simulink model "sliding_car"  (R2017a)
settings: Solver=VariableStepAuto  StartTime=0.0  StopTime=tf  RelTol=1e-3
values from neighbouring files (symbols this model uses):
  R = sys.descrip.syms(end-4)    [load_consts.m]
  sys = kinematic_model(sys)    [load_kin.m]
undefined symbols (not defined in the file or in its folder): a, Cp_1, Cp_2, Fz_1, Fz_2, g, Ic_33, Ii_11, Ii_21, Ii_22, Ii_31, Ii_32, Ii_33, Il_11, Il_21, Il_22, Il_31, Il_32, Il_33, Io_11, Io_21, Io_22, Io_31, Io_32, Io_33, Ir_11, Ir_21, Ir_22, Ir_31, Ir_32, Ir_33, L, Lc, mc, mi, ml, mo, mr, mu_1, mu_2, w, x0
(part 3 of 5)

== matlab function sliding_car/Vehicle/Steering automobile model/Auxiliary matrices/dA_1delta ==
  data: x input; kappa_1 input; kappa_2 input; alpha_1 input; alpha_2 input; w parameter; L parameter; R parameter; dA_1delta output
function dA_1delta = dConstraintMatrix(x, kappa_1, kappa_2, alpha_1, alpha_2, w, L, R)
%DCONSTRAINTMATRIX
%    A_1DELTA = DCONSTRAINTMATRIX(L,R,ALPHA_1,ALPHA_2,DELTA_I,DELTA_O,KAPPA_1,KAPPA_2,THETA,W)

%    This function was generated by the Symbolic Math Toolbox version 7.2.
%    16-Oct-2020 14:33:54
    
    x_pos =  x(1);
    y_pos =  x(2);
    theta =  x(3);

    delta_i = x(4);
    delta_o = x(5);

    phi_i = x(6);
    phi_l = x(7);
    phi_o = x(8);
    phi_r = x(9);

    t2 = tan(delta_i);
    t3 = 1.0./L;
    t4 = t2.*w;
    t5 = L+t4;
    t6 = 1.0./t5;
    t7 = t2.*t6;
    t8 = tan(t7);
    t9 = delta_i+theta;
    t10 = cos(t9);
    t11 = sin(t9);
    t12 = tan(alpha_1);
    t13 = cos(delta_i);
    t14 = sin(delta_i);
    t15 = t14.*w.*(1.0./2.0);
    t16 = kappa_1.*t10.*t12;
    t17 = kappa_1.*t11.*t12;
    t18 = kappa_1.*t12.*(t15-L.*t13);
    t19 = L.*t8;
    t20 = atan(t19);
    t21 = t20+theta;
    t22 = delta_o+theta;
    t23 = tan(alpha_2);
    t24 = L.^2;
    t25 = t8.^2;
    t26 = t24.*t25;
    t27 = t26+1.0;
    t28 = 1.0./sqrt(t27);
    t29 = sin(t21);
    t30 = cos(t22);
    t31 = kappa_2.*t23.*t30;
    t32 = cos(t21);
    t33 = sin(t22);
    t34 = kappa_2.*t23.*t33;
    t35 = cos(delta_o);
    t36 = L.*t35;
    t37 = sin(delta_o);
    t38 = t37.*w.*(1.0./2.0);
    t39 = t36+t38;
    dA_1delta = reshape([0.0, ...
                         0.0, ...
                         t10+t16, ...
                         -t11+t16, ...
                         t31+t32, ...
                         -t29+t31, ...
                         0.0,0.0, ...
                         t11+t17, ...
                         t10+t17, ...
                         t29+t34,t32+t34, ...
                         0.0,0.0, ...
                         t15+t18-L.*t13,t18+L.*t14+t13.*w.*(1.0./2.0), ...
                         -L.*t28-kappa_2.*t23.*t39-L.*t8.*t28.*w.*(1.0./2.0), ...
                         t28.*w.*(-1.0./2.0)-kappa_2.*t23.*t39+t8.*t24.*t28, ...
                         t3.*(t2.^2+1.0).*(L-L.*t8.*w),0.0,0.0,0.0,0.0,0.0, ...
                         -t3.*t5.*t27,0.0,0.0,0.0,0.0,0.0,0.0,0.0,-R, ...
                         0.0,0.0,0.0,0.0,0.0,0.0,0.0,-R,0.0,0.0, ...
                         -t2.*t3.*w-1.0,0.0,0.0,0.0,0.0,0.0, ...
                         1.0,0.0,0.0,0.0,0.0],...
                         [6,9]);

== matlab function sliding_car/Vehicle/Steering automobile model/Ideal, quasi and nonideal efforts/f, f_i, f_ni ==
  data: q input; p input; C_fric input; M input; sqrt_M input; inv_M input; M_12 input; f output; Q input; A_1delta input; Ap_1delta input; C_1delta input; Cp_1delta input; f_i output; f_ni output
function [f, f_i, f_ni] = InputMatrix(q, p, C_fric, M, sqrt_M, inv_M, M_12, Q, A_1delta, Ap_1delta, C_1delta, Cp_1delta)
    %INPUTMATRIX

    %    This function was generated by the Symbolic Math Toolbox version 7.2.
    %    16-Oct-2020 13:53:49

    b_1delta = -Ap_1delta*C_1delta*p;
    
    % Useful constraint    
    B_1delta = A_1delta*M_12;
    
    pB_1delta = pinv(B_1delta);
    
    % ideal constraint
    a = inv_M*Q;
    
    Qc_i = sqrt_M*pB_1delta*(b_1delta - A_1delta*a);    
        
    n = length(pB_1delta);    
    Wc = eye(n) - pB_1delta*B_1delta;
    
    F = sqrt_M*Wc*M_12;
    Qc_ni = F*C_fric;
    
    f = C_1delta.'*Q;
    f_i = -C_1delta.'*M*Cp_1delta*p + C_1delta.'*Qc_i; 
    f_ni = C_1delta.'*Wc*C_fric;
end
